simulink model "SCDalgo_confstate"  (R2019a)
settings: configuration reference "configurationSettings" (kept outside this file)
undefined symbols (not defined in the file or in its folder): SCDalgo_confstate_fp
libraries: dspstat3 x1
settings Model: DataDictionary=SCDalgo_confstate.sldd  Creator=ravensbergen  LastModifiedBy=marceca
settings ConfigSetRef: SourceName=configurationSettings

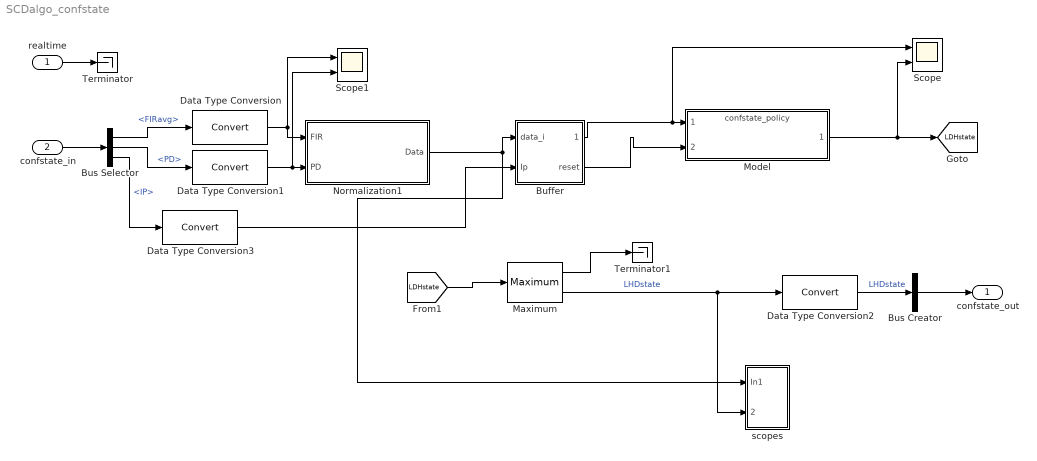
== system SCDalgo_confstate ==
  realtime : Inport  OutDataTypeStr=single  PortDimensions=1  SampleTime=SCDalgo_confstate_fp.timing.dt  Interpolate=off
  confstate_in : Inport  Port=2  OutDataTypeStr=Bus: SCDconfstate_in  PortDimensions=1  SampleTime=SCDalgo_confstate_fp.timing.dt  Interpolate=off  BusOutputAsStruct=on
  Buffer : Subsystem
  Bus Creator : BusCreator  Inputs=1
  Bus Selector : BusSelector  OutputSignals=FIRavg,PD,IP
  Data Type Conversion{,1..3} (4 alike) : DataTypeConversion
  Maximum : dspstat3/Maximum  operation=maximum  fcn=Value and Index  indexBase=One  operateOver=Each column  Dimension=1  InputProcessing=Columns as channels (frame based)  reset=None  roiEnable=off  roiType=Rectangles  roiPortion=Entire ROI  roiOutput=Individual statistics for each ROI  roiFlag=off  roundingMode=Floor  overflowMode=off  accumDataTypeStr=Inherit: Same as product output  accumLastDataTypeStr=Inherit: Same as product output
  Model : ModelReference  ModelNameDialog=confstate_policy.slx  SimulationMode=Normal  ModelReferenceVersion=1.751  SimulationMode=Normal
  Normalization1 : Subsystem
  Scope : Scope  NumInputPorts=2
  Scope1 : Scope  NumInputPorts=2
  Terminator : Terminator
  Terminator1 : Terminator
  scopes : Subsystem
  confstate_out : Outport  OutDataTypeStr=Bus: SCDconfstate_out
  tag scope: LDHstate=global
  wires:
  confstate_in/1 -> Bus Selector/1
  realtime/1 -> Terminator/1
  Buffer/2(reset) -> Model/2
  Normalization1/1(Data) -> scopes/1(In1), Buffer/1(data_i)
  Buffer/1(window_t) -> Scope/1, Model/1
  Model/1 -> Scope/2, [LDHstate]
  Bus Selector/1 -> Data Type Conversion/1  "<FIRavg>"
  Bus Selector/2 -> Data Type Conversion1/1  "<PD>"
  Maximum/2 -> scopes/2(LHDstate), Data Type Conversion2/1  "LHDstate"
  Data Type Conversion/1 -> Scope1/1, Normalization1/1(FIR)
  Data Type Conversion1/1 -> Scope1/2, Normalization1/2(PD)
  Bus Creator/1 -> confstate_out/1
  Data Type Conversion2/1 -> Bus Creator/1  "LHDstate"
  Maximum/1 -> Terminator1/1
  [LDHstate] -> Maximum/1
  Data Type Conversion3/1 -> Buffer/2(Ip)
  Bus Selector/3 -> Data Type Conversion3/1  "<IP>"

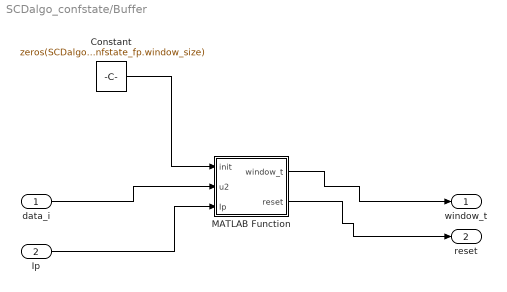
== system SCDalgo_confstate/Buffer ==
  data_i : Inport
  Ip : Inport  Port=2
  Constant : Constant  Value=zeros(SCDalgo_confstate_fp.n_signals, SCDalgo_confstate_fp.window_size)
  MATLAB Function : MATLAB Function  TreatAsAtomicUnit=on
  window_t : Outport
  reset : Outport  Port=2
  wires:
  MATLAB Function/1(window_t) -> window_t/1
  data_i/1 -> MATLAB Function/2(u2)
  MATLAB Function/2(reset) -> reset/1
  Ip/1 -> MATLAB Function/3(Ip)
  Constant/1 -> MATLAB Function/1(init)

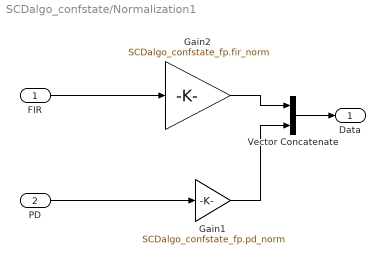
== system SCDalgo_confstate/Normalization1 ==
  FIR : Inport
  PD : Inport  Port=2
  Gain1 : Gain  Gain=SCDalgo_confstate_fp.pd_norm
  Gain2 : Gain  Gain=SCDalgo_confstate_fp.fir_norm
  Vector Concatenate : Concatenate  Mode=Multidimensional array  ConcatenateDimension=2
  Data : Outport
  wires:
  Gain2/1 -> Vector Concatenate/1
  Gain1/1 -> Vector Concatenate/2
  Vector Concatenate/1 -> Data/1
  FIR/1 -> Gain2/1
  PD/1 -> Gain1/1

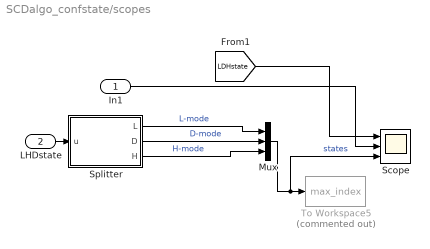
== system SCDalgo_confstate/scopes ==
  In1 : Inport
  LHDstate : Inport  Port=2
  Mux : Mux  Inputs=3
  Scope : Scope  NumInputPorts=3
  Splitter : MATLAB Function  TreatAsAtomicUnit=on
  To Workspace5 : ToWorkspace  Commented=on  VariableName=max_index  SaveFormat=Timeseries  SampleTime=-1
  wires:
  Splitter/2(D) -> Mux/2  "D-mode"
  Splitter/1(L) -> Mux/1  "L-mode"
  Splitter/3(H) -> Mux/3  "H-mode"
  Mux/1 -> Scope/3, To Workspace5/1  "states"
  LHDstate/1 -> Splitter/1(u)
  [LDHstate] -> Scope/1
  In1/1 -> Scope/2

== matlab function SCDalgo_confstate/Buffer/MATLAB Function ==
  data: init input; u2 input; Ip input; window_t output single; reset output; SCDalgo_confstate_tp parameter
function [window_t, reset] = buffer(init,u2, Ip, SCDalgo_confstate_tp)
%#codegen
[window_t, reset] = buffer_func(init,u2, Ip, SCDalgo_confstate_tp);

== matlab function SCDalgo_confstate/scopes/Splitter ==
  data: u input; L output; D output; H output
function [L,D,H]  = splitter(u)

L = u == 1;
D = u == 2;
H = u == 3;
